simulink model "QPSK_modulator"  (R2025b)
settings: Solver=VariableStepAuto  StartTime=0.0  StopTime=50e-6  RelTol=1e-3
libraries: commfilt2 x2, dspsigops x2, dspsrcs4 x1
settings Model: Creator=bobyc  LastModifiedBy=bobyc

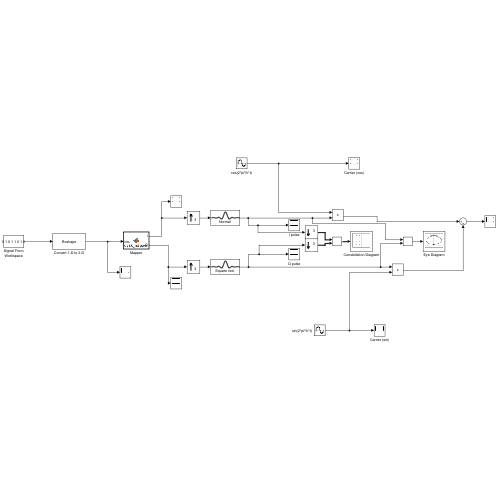
[thumbnail: Simulink's stored preview of the top-level diagram]
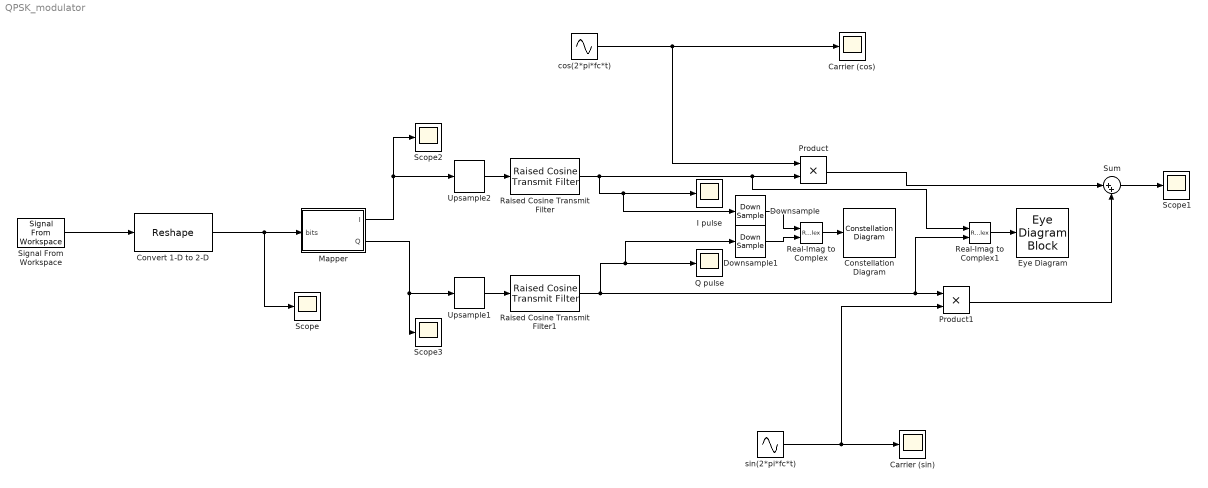
== system QPSK_modulator ==
  Carrier (cos) : Scope
      settings: ActiveDisplayYMinimum=-1.1152961855777177  ActiveDisplayYMaximum=1.0387593761338962  DataLoggingVariableName=ScopeData5
  Carrier (sin) : Scope
      settings: ActiveDisplayYMinimum=-1.1566922028256013  ActiveDisplayYMaximum=1.0017628526691322  DataLoggingVariableName=ScopeData6
  Constellation Diagram : ConstellationDiagram  WindowPosition=[146.000000,59.000000,600.000000,552.000000,]  ScopeFrameLocation=window  EnableMeasurements=on
  Convert 1-D to 2-D : Reshape  OutputDimensionality=Customize  OutputDimensions=[2 1]
  Downsample : DownSample  N=3  AllowArbitraryFixedInput=on
  Downsample1 : DownSample  N=3  AllowArbitraryFixedInput=on
  Eye Diagram : EyeDiagramBlock  WindowPosition=[281.000000,90.000000,800.000000,500.000000,]  ScopeFrameLocation=window
  I pulse : Scope
      settings: ActiveDisplayYMinimum=-1.4415795214515996  ActiveDisplayYMaximum=1.2384002174819631  DataLoggingVariableName=ScopeData9
  Mapper : MATLAB Function  TreatAsAtomicUnit=on
  Product : Product
  Product1 : Product
  Q pulse : Scope
      settings: ActiveDisplayYMinimum=-1.8851379276580049  ActiveDisplayYMaximum=1.0349047296099532  DataLoggingVariableName=ScopeData2
  Raised Cosine Transmit Filter : commfilt2/Raised Cosine Transmit Filter  filtType=Normal  R=0.35  filtSpan=4  N=3  filterGain=1  RateOptions=Allow multirate processing  framing=Mute  checkCoeff=off  variableName=rcTxFilt  checkGain=Normalized  sampMode=Mute  saveAsFlag=0  currentFiltSpan=10  D=(10)/2  launchFVT=on  roundingMode=Floor  overflowMode=off  coeffDataTypeStr=Inherit: Same word length as input  coeffMin=[]  coeffMax=[]  coeffLastDataTypeStr=Inherit: Same word length as input  outputDataTypeStr=Inherit: Same as accumulator  outputMin=[]  outputMax=[]  outputLastDataTypeStr=Inherit: Same as accumulator
  Raised Cosine Transmit Filter1 : commfilt2/Raised Cosine Transmit Filter  filtType=Square root  R=0.35  filtSpan=4  N=3  filterGain=1  RateOptions=Allow multirate processing  framing=Mute  checkCoeff=off  variableName=rcTxFilt1  checkGain=Normalized  sampMode=Mute  saveAsFlag=0  currentFiltSpan=10  D=(10)/2  launchFVT=on  roundingMode=Floor  overflowMode=off  coeffDataTypeStr=Inherit: Same word length as input  coeffMin=[]  coeffMax=[]  coeffLastDataTypeStr=Inherit: Same word length as input  outputDataTypeStr=Inherit: Same as accumulator  outputMin=[]  outputMax=[]  outputLastDataTypeStr=Inherit: Same as accumulator
  Real-Imag to Complex : RealImagToComplex
  Real-Imag to Complex1 : RealImagToComplex
  Scope{,1..3} (4 alike) : Scope
      Scope settings: ActiveDisplayYMinimum=-7.4585395124822469  ActiveDisplayYMaximum=6.7511085062467551
      Scope1 settings: ActiveDisplayYMinimum=-2.4774137252708153  ActiveDisplayYMaximum=1.6929863682080144
      Scope2 settings: ActiveDisplayYMinimum=-1.25  ActiveDisplayYMaximum=1.25  DataLoggingVariableName=ScopeData3
      Scope3 settings: ActiveDisplayYMinimum=-1.25  ActiveDisplayYMaximum=1.25  DataLoggingVariableName=ScopeData4
  Signal From Workspace : dspsrcs4/Signal From Workspace  X=[1 0 1 1 0 1 1 0 1 0 1 1 0 1 0 0 1 1 0 0 1 0]  Ts=1/1000000  nsamps=2  OutputAfterFinalValue=Setting to zero  ignoreOrWarnInputAndFrameLengths=off  OutputFrames=off
  Sum : Sum  Inputs=|++
  Upsample1 : dspsigops/Upsample  FactorSource=Dialog parameter  N=3  Nmax=16  phase=0  InputProcessing=Columns as channels (frame based)  RateOptions=Enforce single-rate processing  ic=0  mode=Unused parameter value
  Upsample2 : dspsigops/Upsample  FactorSource=Dialog parameter  N=3  Nmax=16  phase=0  InputProcessing=Columns as channels (frame based)  RateOptions=Enforce single-rate processing  ic=0  mode=Unused parameter value
  cos(2*pi*fc*t) : Sin  Frequency=2*pi*30000000  Phase=pi/2  SampleTime=2e-9
  sin(2*pi*fc*t) : Sin  Frequency=2*pi*30000000  Phase=pi  SampleTime=2e-9
  wires:
  Upsample1/1 -> Raised Cosine Transmit Filter1/1
  Upsample2/1 -> Raised Cosine Transmit Filter/1
  Mapper/1(I) -> Scope2/1, Upsample2/1
  Mapper/2(Q) -> Scope3/1, Upsample1/1
  Convert 1-D to 2-D/1 -> Scope/1, Mapper/1(bits)
  Raised Cosine Transmit Filter/1 -> Downsample/1, I pulse/1, Real-Imag to Complex1/1, Product/2
  cos(2*pi*fc*t)/1 -> Product/1, Carrier (cos)/1
  Product/1 -> Sum/1
  sin(2*pi*fc*t)/1 -> Product1/2, Carrier (sin)/1
  Product1/1 -> Sum/2
  Raised Cosine Transmit Filter1/1 -> Downsample1/1, Q pulse/1, Real-Imag to Complex1/2, Product1/1
  Sum/1 -> Scope1/1
  Signal From Workspace/1 -> Convert 1-D to 2-D/1
  Real-Imag to Complex/1 -> Constellation Diagram/1
  Downsample1/1 -> Real-Imag to Complex/2
  Downsample/1 -> Real-Imag to Complex/1
  Real-Imag to Complex1/1 -> Eye Diagram/1

== matlab function QPSK_modulator/Mapper ==
  data: bits input; I output; Q output
function [I, Q] = qpsk_mapper(bits)
%#codegen
if isequal(bits,[0;0])
    I = 1;  Q = 1;
elseif isequal(bits,[0;1])
    I = -1; Q = 1;
elseif isequal(bits,[1;1])
    I = -1; Q = -1;
else % [1;0]
    I = 1;  Q = -1;
end
end
